simulink model "simmodel"  (R2014b)
settings: Solver=ode3  StartTime=0.0  StopTime=50  FixedStep=dt  RelTol=1e-3
values from neighbouring files (symbols this model uses):
  dt = 0.01    [expathplan.m]
  origin = [0, 0, 0]    [initdynprog.m]
  Path = []    [expathplan.m]    (also in initdynprog.m = zeros(1,8*maxarc))
  sPath = 0    [initdynprog.m]
  u0 = [0 0 1]    [expathplan.m]
  x0 = [8.5 7 0]    [expathplan.m]
undefined symbols (not defined in the file or in its folder): car
settings Model: Creator=schilgeo  LastModifiedBy=schilgeo
settings DebuggingCC: UnderspecifiedInitializationDetection=Classic  MergeDetectMultiDrivingBlocksExec=none
settings RTWCC: GenCodeOnly=on

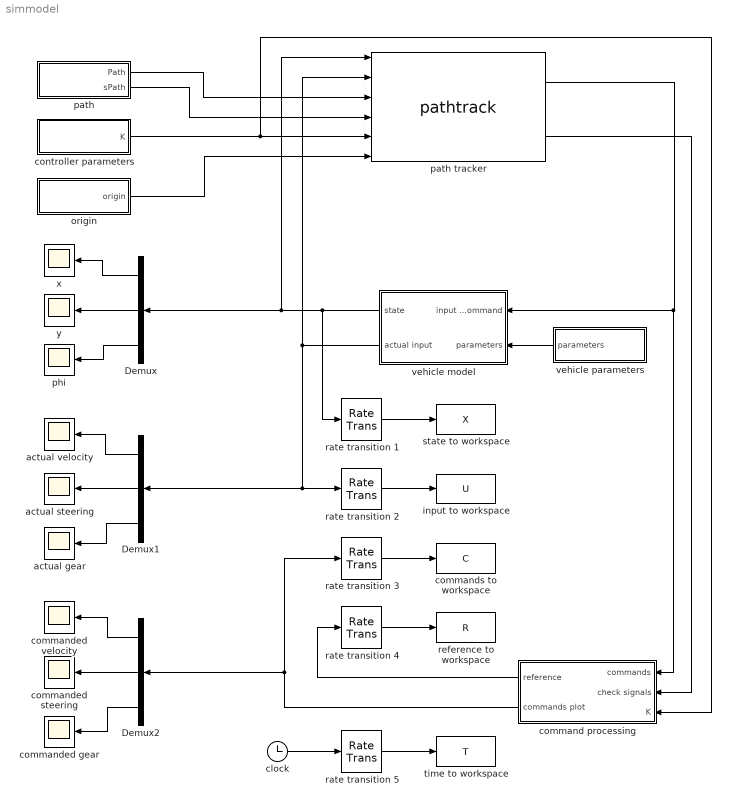
== system simmodel ==
  Demux : Demux  Outputs=3
  Demux1 : Demux  Outputs=3
  Demux2 : Demux  Outputs=3
  actual gear : Scope
      settings: SaveName=ScopeData3
  actual steering : Scope
      settings: SaveName=ScopeData6
  actual velocity : Scope
      settings: SaveName=ScopeData5
  clock : Clock
  command processing : Subsystem
  commanded gear : Scope
      settings: SaveName=ScopeData4
  commanded steering : Scope
      settings: TimeRange=1  YMin=0  YMax=1  SaveName=ScopeData8
  commanded velocity : Scope
      settings: SaveName=ScopeData7
  commands to workspace : ToWorkspace  VariableName=C  SampleTime=0.1
  controller parameters : Subsystem
  input to workspace : ToWorkspace  VariableName=U  SampleTime=0.1
  origin : Subsystem
  path : Subsystem
  path tracker : S-Function  FunctionName=pathtrack  EnableBusSupport=off
      mask Display:
      | port_label('output', 1, 'commands')
      | port_label('output', 2, 'check signals')
      | port_label('input', 1, 'x,y,phi')
      | port_label('input', 2, 'abs(v),delta,gear')
      | port_label('input', 3, 'Path')
      | port_label('input', 4, 'sPath')
      | port_label('input', 5, 'parameters')
      | port_label('input', 6, 'origin')
  phi : Scope
      settings: SaveName=ScopeData2
  rate transition {1..5} (5 alike) : RateTransition  OutPortSampleTime=0.1
  reference to workspace : ToWorkspace  VariableName=R  SampleTime=0.1
  state to workspace : ToWorkspace  VariableName=X  SampleTime=0.1
  time to workspace : ToWorkspace  VariableName=T  SampleTime=0.1
  vehicle model : Subsystem
  vehicle parameters : Subsystem
  x : Scope
  y : Scope
  wires:
  clock/1 -> rate transition 5/1
  vehicle model/1(state) -> rate transition 1/1, path tracker/1, Demux/1
  Demux/3 -> phi/1
  Demux/2 -> y/1
  Demux/1 -> x/1
  Demux1/2 -> actual steering/1
  Demux2/2 -> commanded steering/1
  vehicle parameters/1(parameters) -> vehicle model/2(parameters)
  path tracker/1 -> command processing/1(commands), vehicle model/1(input command)
  Demux2/1 -> commanded velocity/1
  Demux2/3 -> commanded gear/1
  Demux1/3 -> actual gear/1
  Demux1/1 -> actual velocity/1
  path/1(Path) -> path tracker/3
  path/2(sPath) -> path tracker/4
  controller parameters/1(K) -> command processing/3(K), path tracker/5
  vehicle model/2(actual input) -> rate transition 2/1, Demux1/1, path tracker/2
  rate transition 1/1 -> state to workspace/1
  rate transition 2/1 -> input to workspace/1
  rate transition 3/1 -> commands to workspace/1
  rate transition 5/1 -> time to workspace/1
  origin/1(origin) -> path tracker/6
  path tracker/2 -> command processing/2(check signals)
  command processing/2(commands plot) -> Demux2/1, rate transition 3/1
  rate transition 4/1 -> reference to workspace/1
  command processing/1(reference) -> rate transition 4/1

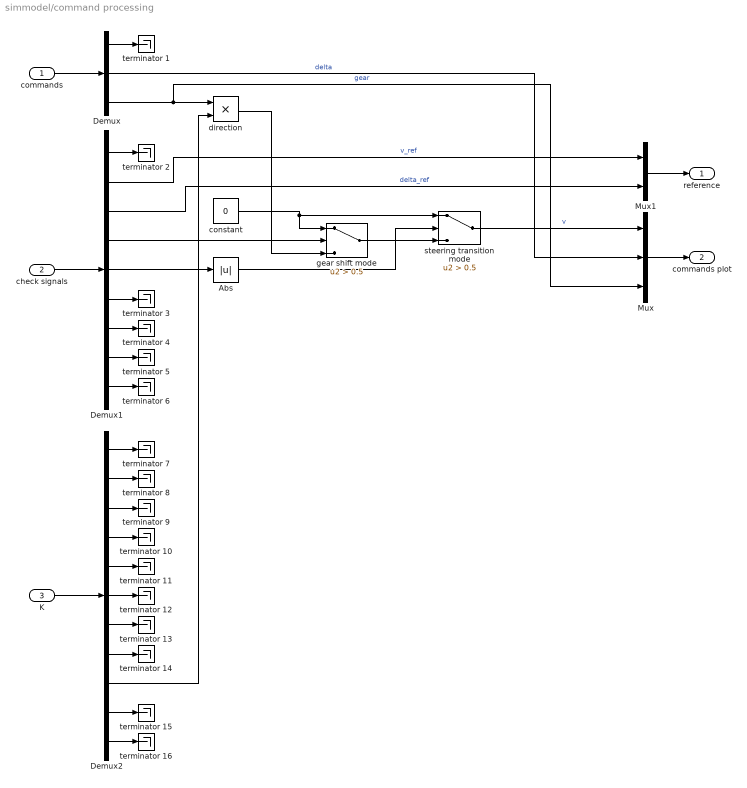
== system simmodel/command processing ==
  commands : Inport
  check signals : Inport  Port=2
  K : Inport  Port=3
  Abs : Abs
  Demux : Demux  Outputs=3
  Demux1 : Demux  Outputs=9
  Demux2 : Demux  Outputs=11
  Mux : Mux  Inputs=3
  Mux1 : Mux  Inputs=2
  constant : Constant  Value=0
  direction : Product  Inputs=**
  gear shift mode : Switch  Criteria=u2 > Threshold  Threshold=0.5
  steering transition mode : Switch  Criteria=u2 > Threshold  Threshold=0.5
  terminator {1..16} (16 alike) : Terminator
  reference : Outport
  commands plot : Outport  Port=2
  wires:
  commands/1 -> Demux/1
  check signals/1 -> Demux1/1
  Demux1/4 -> gear shift mode/2
  constant/1 -> steering transition mode/1, gear shift mode/1
  Demux1/5 -> Abs/1
  Abs/1 -> steering transition mode/2
  gear shift mode/1 -> steering transition mode/3
  K/1 -> Demux2/1
  Demux2/9 -> direction/2
  Demux/3 -> Mux/3, direction/1  "gear"
  direction/1 -> gear shift mode/3
  Mux/1 -> commands plot/1
  steering transition mode/1 -> Mux/1  "v"
  Demux/2 -> Mux/2  "delta"
  Mux1/1 -> reference/1
  Demux1/3 -> Mux1/2  "delta_ref"
  Demux1/2 -> Mux1/1  "v_ref"
  Demux/1 -> terminator 1/1
  Demux1/1 -> terminator 2/1
  Demux1/6 -> terminator 3/1
  Demux1/7 -> terminator 4/1
  Demux1/8 -> terminator 5/1
  Demux1/9 -> terminator 6/1
  Demux2/1 -> terminator 7/1
  Demux2/2 -> terminator 8/1
  Demux2/3 -> terminator 9/1
  Demux2/4 -> terminator 10/1
  Demux2/5 -> terminator 11/1
  Demux2/6 -> terminator 12/1
  Demux2/7 -> terminator 13/1
  Demux2/8 -> terminator 14/1
  Demux2/10 -> terminator 15/1
  Demux2/11 -> terminator 16/1

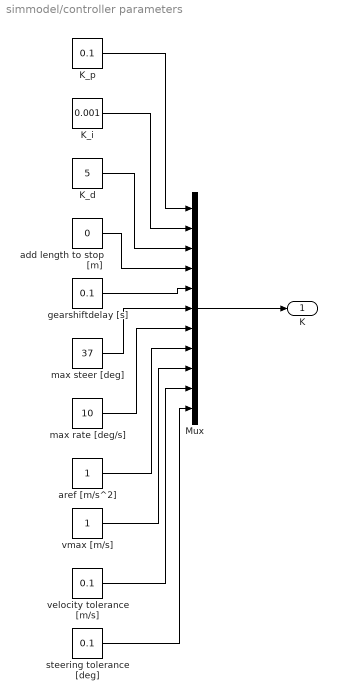
== system simmodel/controller parameters ==
  K_d : Constant  Value=5
  K_i : Constant  Value=0.001
  K_p : Constant  Value=0.1
  Mux : Mux  Inputs=11
  add length to stop [m] : Constant  Value=0
  aref [m/s^2] : Constant
  gearshiftdelay [s] : Constant  Value=0.1
  max rate [deg/s] : Constant  Value=10
  max steer [deg] : Constant  Value=37
  steering tolerance [deg] : Constant  Value=0.1
  velocity tolerance [m/s] : Constant  Value=0.1
  vmax [m/s] : Constant
  K : Outport
  wires:
  Mux/1 -> K/1
  gearshiftdelay [s]/1 -> Mux/5
  velocity tolerance [m/s]/1 -> Mux/10
  aref [m/s^2]/1 -> Mux/8
  max rate [deg/s]/1 -> Mux/7
  max steer [deg]/1 -> Mux/6
  K_p/1 -> Mux/1
  K_i/1 -> Mux/2
  K_d/1 -> Mux/3
  add length to stop [m]/1 -> Mux/4
  steering tolerance [deg]/1 -> Mux/11
  vmax [m/s]/1 -> Mux/9

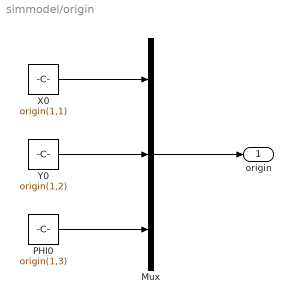
== system simmodel/origin ==
  Mux : Mux  Inputs=3
  PHI0 : Constant  Value=origin(1,3)
  X0 : Constant  Value=origin(1,1)
  Y0 : Constant  Value=origin(1,2)
  origin : Outport
  wires:
  Mux/1 -> origin/1
  X0/1 -> Mux/1
  PHI0/1 -> Mux/3
  Y0/1 -> Mux/2

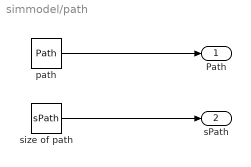
== system simmodel/path ==
  path : Constant  Value=Path
  size of path : Constant  Value=sPath
  Path : Outport
  sPath : Outport  Port=2
  wires:
  path/1 -> Path/1
  size of path/1 -> sPath/1

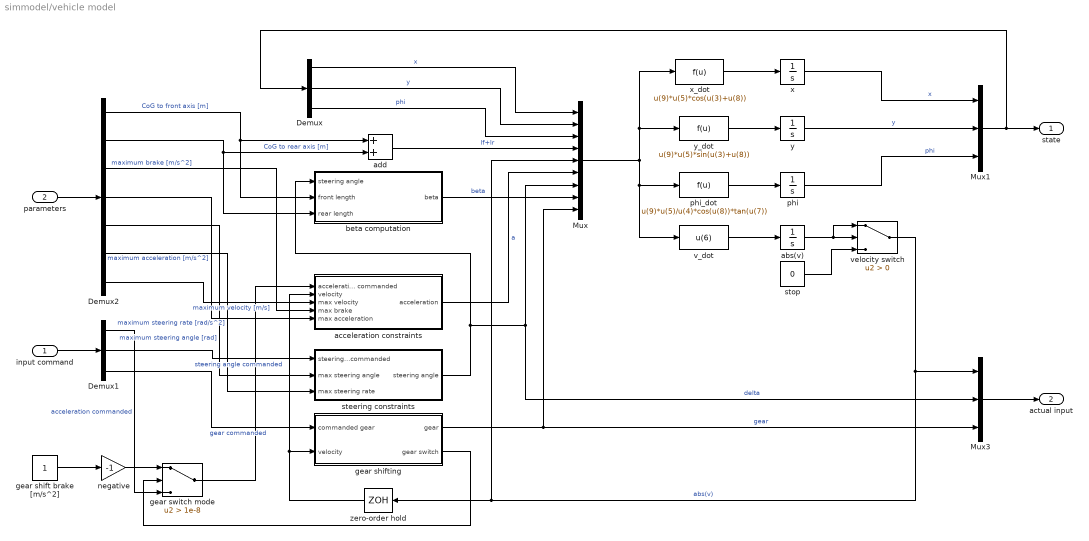
== system simmodel/vehicle model ==
  input command : Inport
  parameters : Inport  Port=2
  Demux : Demux  Outputs=3
  Demux1 : Demux  Outputs=3
  Demux2 : Demux  Outputs=7
  Mux : Mux  Inputs=9
  Mux1 : Mux  Inputs=3
  Mux3 : Mux  Inputs=3
  abs(v) : Integrator  InitialCondition=u0(1)  LimitOutput=on  UpperSaturationLimit=100  LowerSaturationLimit=0
  acceleration constraints : Subsystem
  add : Sum
  beta computation : Subsystem
  gear shift brake [m/s^2] : Constant
  gear shifting : Subsystem
  gear switch mode : Switch  Criteria=u2 > Threshold  Threshold=1e-8
  negative : Gain  Gain=-1
  phi : Integrator  InitialCondition=x0(3)
  phi_dot : Fcn  Expr=u(9)*u(5)/u(4)*cos(u(8))*tan(u(7))
  steering constraints : Subsystem
  stop : Constant  Value=0
  v_dot : Fcn  Expr=u(6)
  velocity switch : Switch  Criteria=u2 > Threshold
  x : Integrator  InitialCondition=x0(1)
  x_dot : Fcn  Expr=u(9)*u(5)*cos(u(3)+u(8))
  y : Integrator  InitialCondition=x0(2)
  y_dot : Fcn  Expr=u(9)*u(5)*sin(u(3)+u(8))
  zero-order hold : ZeroOrderHold  SampleTime=dt
  state : Outport
  actual input : Outport  Port=2
  wires:
  input command/1 -> Demux1/1
  Demux/1 -> Mux/1  "x"
  Demux/3 -> Mux/3  "phi"
  Demux/2 -> Mux/2  "y"
  beta computation/1(beta) -> Mux/8  "beta"
  Mux1/1 -> state/1, Demux/1
  x_dot/1 -> x/1
  v_dot/1 -> abs(v)/1
  phi_dot/1 -> phi/1
  y_dot/1 -> y/1
  phi/1 -> Mux1/3  "phi"
  x/1 -> Mux1/1  "x"
  y/1 -> Mux1/2  "y"
  steering constraints/1(steering angle) -> beta computation/1(steering angle), Mux3/2, Mux/7  "delta"
  parameters/1 -> Demux2/1
  Demux1/2 -> steering constraints/1(steering commanded)  "steering angle commanded"
  Demux1/1 -> gear switch mode/3  "acceleration commanded"
  Demux2/3 -> acceleration constraints/4(max brake)  "maximum brake [m/s^2]"
  Demux2/4 -> acceleration constraints/5(max acceleration)  "maximum acceleration [m/s^2]"
  Demux2/5 -> steering constraints/2(max steering angle)  "maximum steering angle [rad]"
  Demux2/6 -> steering constraints/3(max steering rate)  "maximum steering rate [rad/s^2]"
  Demux2/1 -> add/1, beta computation/2(front length)  "CoG to front axis [m]"
  Demux2/2 -> add/2, beta computation/3(rear length)  "CoG to rear axis [m]"
  add/1 -> Mux/4  "lf+lr"
  Demux1/3 -> gear shifting/1(commanded gear)  "gear commanded"
  gear shifting/1(gear) -> Mux/9, Mux3/3  "gear"
  Mux/1 -> x_dot/1, y_dot/1, v_dot/1, phi_dot/1
  zero-order hold/1 -> acceleration constraints/2(velocity), gear shifting/2(velocity)
  gear shifting/2(gear switch) -> gear switch mode/2
  gear switch mode/1 -> acceleration constraints/1(acceleration commanded)
  acceleration constraints/1(acceleration) -> Mux/6  "a"
  Demux2/7 -> acceleration constraints/3(max velocity)  "maximum velocity [m/s]"
  gear shift brake [m/s^2]/1 -> negative/1
  Mux3/1 -> actual input/1
  abs(v)/1 -> velocity switch/1, velocity switch/2
  stop/1 -> velocity switch/3
  velocity switch/1 -> Mux/5, zero-order hold/1, Mux3/1  "abs(v)"
  negative/1 -> gear switch mode/1

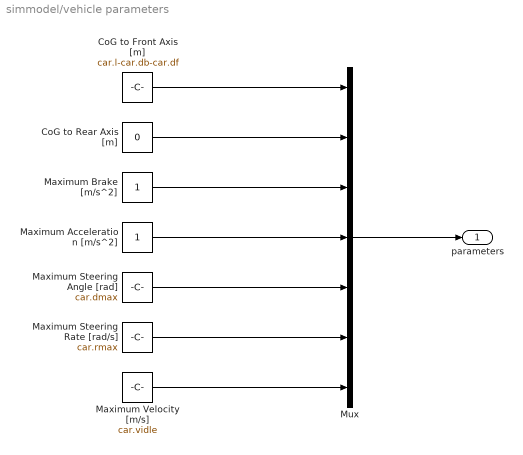
== system simmodel/vehicle parameters ==
  CoG to Front Axis [m] : Constant  Value=car.l-car.db-car.df
  CoG to Rear Axis [m] : Constant  Value=0
  Maximum Acceleration [m/s^2] : Constant
  Maximum Brake [m/s^2] : Constant
  Maximum Steering Angle [rad] : Constant  Value=car.dmax
  Maximum Steering Rate [rad/s] : Constant  Value=car.rmax
  Maximum Velocity [m/s] : Constant  Value=car.vidle
  Mux : Mux  Inputs=7
  parameters : Outport
  wires:
  Mux/1 -> parameters/1
  Maximum Steering Angle [rad]/1 -> Mux/5
  Maximum Steering Rate [rad/s]/1 -> Mux/6
  CoG to Front Axis [m]/1 -> Mux/1
  CoG to Rear Axis [m]/1 -> Mux/2
  Maximum Brake [m/s^2]/1 -> Mux/3
  Maximum Acceleration [m/s^2]/1 -> Mux/4
  Maximum Velocity [m/s]/1 -> Mux/7

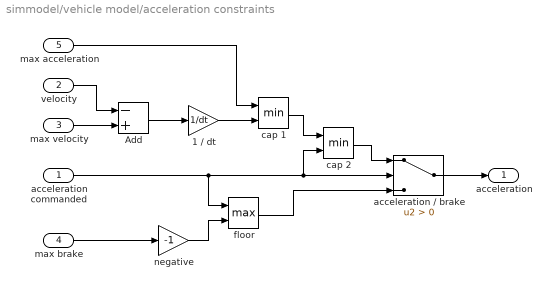
== system simmodel/vehicle model/acceleration constraints ==
  acceleration commanded : Inport
  velocity : Inport  Port=2
  max velocity : Inport  Port=3
  max brake : Inport  Port=4
  max acceleration : Inport  Port=5
  1 / dt : Gain  Gain=1/dt
  Add : Sum  Inputs=-+
  acceleration / brake : Switch  Criteria=u2 > Threshold
  cap 1 : MinMax  Inputs=2
  cap 2 : MinMax  Inputs=2
  floor : MinMax  Function=max  Inputs=2
  negative : Gain  Gain=-1
  acceleration : Outport
  wires:
  max acceleration/1 -> cap 1/1
  max brake/1 -> negative/1
  acceleration commanded/1 -> floor/1, cap 2/2, acceleration / brake/2
  cap 2/1 -> acceleration / brake/1
  max velocity/1 -> Add/2
  velocity/1 -> Add/1
  Add/1 -> 1 / dt/1
  1 / dt/1 -> cap 1/2
  negative/1 -> floor/2
  acceleration / brake/1 -> acceleration/1
  floor/1 -> acceleration / brake/3
  cap 1/1 -> cap 2/1

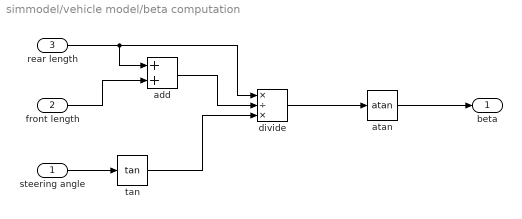
== system simmodel/vehicle model/beta computation ==
  steering angle : Inport
  front length : Inport  Port=2
  rear length : Inport  Port=3
  add : Sum
  atan : Trigonometry  Operator=atan
  divide : Product  Inputs=*/*
  tan : Trigonometry  Operator=tan
  beta : Outport
  wires:
  rear length/1 -> divide/1, add/1
  front length/1 -> add/2
  steering angle/1 -> tan/1
  tan/1 -> divide/3
  add/1 -> divide/2
  divide/1 -> atan/1
  atan/1 -> beta/1

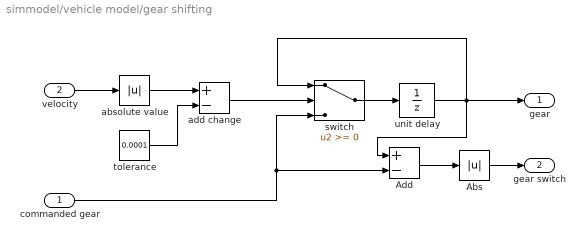
== system simmodel/vehicle model/gear shifting ==
  commanded gear : Inport
  velocity : Inport  Port=2
  Abs : Abs
  Add : Sum  Inputs=+-
  absolute value : Abs
  add change : Sum  Inputs=+-
  switch : Switch
  tolerance : Constant  Value=0.0001
  unit delay : UnitDelay  InitialCondition=u0(3)  SampleTime=-1
  gear : Outport
  gear switch : Outport  Port=2
  wires:
  velocity/1 -> absolute value/1
  switch/1 -> unit delay/1
  absolute value/1 -> add change/1
  tolerance/1 -> add change/2
  add change/1 -> switch/2
  commanded gear/1 -> Add/2, switch/3
  unit delay/1 -> Add/1, switch/1, gear/1
  Add/1 -> Abs/1
  Abs/1 -> gear switch/1

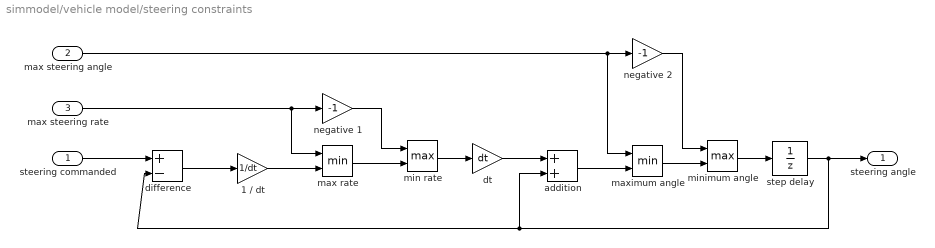
== system simmodel/vehicle model/steering constraints ==
  steering commanded : Inport
  max steering angle : Inport  Port=2
  max steering rate : Inport  Port=3
  " negative 2" : Gain  Gain=-1
  1 / dt : Gain  Gain=1/dt
  addition : Sum
  difference : Sum  Inputs=+-
  dt : Gain  Gain=dt
  max rate : MinMax  Inputs=2
  maximum angle : MinMax  Inputs=2
  min rate : MinMax  Function=max  Inputs=2
  minimum angle : MinMax  Function=max  Inputs=2
  negative 1 : Gain  Gain=-1
  step delay : UnitDelay  InitialCondition=u0(2)  SampleTime=-1
  steering angle : Outport
  wires:
  max steering angle/1 -> maximum angle/1, " negative 2"/1
  maximum angle/1 -> minimum angle/2
  " negative 2"/1 -> minimum angle/1
  negative 1/1 -> min rate/1
  max rate/1 -> min rate/2
  max steering rate/1 -> max rate/1, negative 1/1
  min rate/1 -> dt/1
  difference/1 -> 1 / dt/1
  steering commanded/1 -> difference/1
  1 / dt/1 -> max rate/2
  minimum angle/1 -> step delay/1
  dt/1 -> addition/1
  addition/1 -> maximum angle/2
  step delay/1 -> difference/2, addition/2, steering angle/1
